simulink model "Pacemaker_model_assgn2_2019a"  (R2019a)
settings: Solver=FixedStepAuto  StartTime=0.0  StopTime=inf  FixedStep=1e-3  RelTol=1e-3  EnableMultiTasking=on
undefined symbols (not defined in the file): D0, D1, D10, D11, D12, D13, D2, D3, D4, D5, D6, D7, D8, D9, PTA0, PTA1, PTA2, PTB23, PTB9, PTC16, PTC17, PTC2, PTC3, PTC4, PTD0, PTD1, PTD2, PTD3
libraries: frdmk64flib x21, etargetslib x15, dspstat3 x1
settings Model: ExtModeTrigDuration=5  Creator=dr_pa  LastModifiedBy=dr_pa
settings SolverCC: ConcurrentTasks=on
settings OptimizationCC: EnhancedBackFolding=on  PassReuseOutputArgsAs=Individual arguments  MaxStackSize=64  OptimizeBlockOrder=speed  DifferentSizesBufferReuse=on  OptimizationCustomize=off
settings DebuggingCC: ParameterTunabilityLossMsg=error
settings HardwareCC: ProdBitPerPointer=32  ProdBitPerSizeT=32  ProdBitPerPtrDiffT=32  ProdLargestAtomicInteger=Long  ProdLargestAtomicFloat=Double  ProdWordSize=32  ProdHWDeviceType=ARM Compatible->ARM Cortex
settings SFSimCC: MATLABDynamicMemAlloc=off
settings RTWCC: SystemTargetFile=ert.tlc  HardwareBoard=NXP FRDM-K64F  TLCOptions="-aInlineSetEventsForThisBaseRateFcn=TLC_FALSE -aSuppressMultiTaskScheduler=TLC_FALSE  -aRateBasedStepFcn=0"  TemplateMakefile=ert_default_tmf  GenerateReport=on  Toolchain=GNU Tools for ARM Embedded Processors  BuildConfiguration=Faster Runs  IncludeHyperlinkInReport=on  LaunchReport=on  GenerateTraceInfo=on  GenerateTraceReport=on  GenerateTraceReportSl=on  GenerateTraceReportSf=on  GenerateTraceReportEml=on
settings CodeAppCC: ForceParamTrailComments=on  IgnoreCustomStorageClasses=off  OperatorAnnotations=on  SimulinkDataObjDesc=on  SFDataObjDesc=on  InsertBlockDesc=on

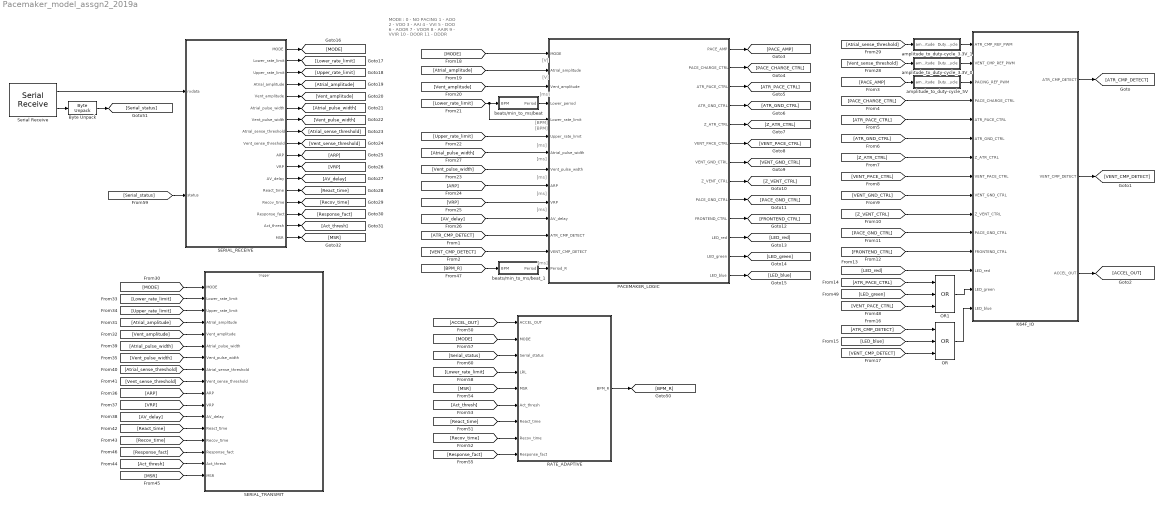
== system Pacemaker_model_assgn2_2019a ==
  note: [V]
  note: MODE :
      | 0 - NO PACING
      | 1 - AOO
      | 2 - VOO
      | 3 - AAI
      | 4 - VVI
      | 5 - DOO
      | 6 - AOOR
      | 7 - VOOR
      | 8 - AAIR
      | 9 - VVIR
      | 10 - DOOR
      | 11 - DDDR
  note: [V]
  note: [ms]
  note: [BPM]
  note: [BPM]
  note: [ms]
  note: [ms]
  note: [ms]
  note: [ms]
  note: [ms]
  note: [ms]
  Byte Unpack : etargetslib/Byte Unpack  dimensions={[1]}  datatypes={'uint8'}  byteAlign=1
      settings: SourceProductName=MATLAB Coder
  K64F_IO : Subsystem
  OR : Logic  Operator=OR  Inputs=3  IconShape=distinctive  AllPortsSameDT=off  OutDataTypeStr=boolean
  OR1 : Logic  Operator=OR  Inputs=3  IconShape=distinctive  AllPortsSameDT=off  OutDataTypeStr=boolean
  PACEMAKER_LOGIC : Stateflow chart  BlockKeywords=__PRM__SERIALIZED__DATA__:Stateflow Chart,Stateflow Diagram  TreatAsAtomicUnit=on
  RATE_ADAPTIVE : Subsystem
  SERIAL_RECEIVE : Stateflow chart  BlockKeywords=__PRM__SERIALIZED__DATA__:Stateflow Chart,Stateflow Diagram  TreatAsAtomicUnit=on
  SERIAL_TRANSMIT : Subsystem  TreatAsAtomicUnit=on
  Serial Receive : frdmk64flib/Serial Receive  SCIModule=0  Baudrate=uint32(9600)  Parity=None  StopBits=1  HardwareFlowControl=None  ByteOrder=LittleEndian  DataType=uint8  DataLength=56  BlockingMode=off  OutputStatus=on  SampleTime=-1
      settings: SourceProductName=Simulink Coder Support Package for NXP FRDM-K64F Board
  amplitude_to_duty-cycle_3.3V_0 : Subsystem
  amplitude_to_duty-cycle_3.3V_1 : Subsystem
  amplitude_to_duty-cycle_5V : Subsystem
  beats/min_to_ms/beat : Subsystem
  beats/min_to_ms/beat_1 : Subsystem
  wires:
  amplitude_to_duty-cycle_5V/1(Duty Cycle) -> K64F_IO/3(PACING_REF_PWM)
  beats/min_to_ms/beat/1(Period) -> PACEMAKER_LOGIC/4(Lower_period)
  amplitude_to_duty-cycle_3.3V_0/1(Duty Cycle) -> K64F_IO/2(VENT_CMP_REF_PWM)
  amplitude_to_duty-cycle_3.3V_1/1(Duty Cycle) -> K64F_IO/1(ATR_CMP_REF_PWM)
  K64F_IO/1(ATR_CMP_DETECT) -> [ATR_CMP_DETECT]
  [ATR_CMP_DETECT] -> PACEMAKER_LOGIC/12(ATR_CMP_DETECT)
  K64F_IO/2(VENT_CMP_DETECT) -> [VENT_CMP_DETECT]
  [VENT_CMP_DETECT] -> PACEMAKER_LOGIC/13(VENT_CMP_DETECT)
  K64F_IO/3(ACCEL_OUT) -> [ACCEL_OUT]
  RATE_ADAPTIVE/1(BPM_R) -> [BPM_R]
  OR/1 -> K64F_IO/15(LED_blue)
  Serial Receive/1 -> SERIAL_RECEIVE/1(rxdata)
  Serial Receive/2 -> Byte Unpack/1
  PACEMAKER_LOGIC/1(PACE_AMP) -> [PACE_AMP]
  [PACE_AMP] -> amplitude_to_duty-cycle_5V/1(amplitude)
  PACEMAKER_LOGIC/2(PACE_CHARGE_CTRL) -> [PACE_CHARGE_CTRL]
  [PACE_CHARGE_CTRL] -> K64F_IO/4(PACE_CHARGE_CTRL)
  [ATR_PACE_CTRL] -> K64F_IO/5(ATR_PACE_CTRL)
  PACEMAKER_LOGIC/4(ATR_GND_CTRL) -> [ATR_GND_CTRL]
  [ATR_GND_CTRL] -> K64F_IO/6(ATR_GND_CTRL)
  [Z_ATR_CTRL] -> K64F_IO/7(Z_ATR_CTRL)
  PACEMAKER_LOGIC/5(Z_ATR_CTRL) -> [Z_ATR_CTRL]
  PACEMAKER_LOGIC/6(VENT_PACE_CTRL) -> [VENT_PACE_CTRL]
  [VENT_PACE_CTRL] -> K64F_IO/8(VENT_PACE_CTRL)
  PACEMAKER_LOGIC/7(VENT_GND_CTRL) -> [VENT_GND_CTRL]
  [VENT_GND_CTRL] -> K64F_IO/9(VENT_GND_CTRL)
  PACEMAKER_LOGIC/8(Z_VENT_CTRL) -> [Z_VENT_CTRL]
  [Z_VENT_CTRL] -> K64F_IO/10(Z_VENT_CTRL)
  PACEMAKER_LOGIC/9(PACE_GND_CTRL) -> [PACE_GND_CTRL]
  [PACE_GND_CTRL] -> K64F_IO/11(PACE_GND_CTRL)
  [FRONTEND_CTRL] -> K64F_IO/12(FRONTEND_CTRL)
  PACEMAKER_LOGIC/10(FRONTEND_CTRL) -> [FRONTEND_CTRL]
  PACEMAKER_LOGIC/11(LED_red) -> [LED_red]
  [LED_red] -> K64F_IO/13(LED_red)
  PACEMAKER_LOGIC/12(LED_green) -> [LED_green]
  PACEMAKER_LOGIC/13(LED_blue) -> [LED_blue]
  [LED_blue] -> OR/2
  [ATR_CMP_DETECT] -> OR/1
  [VENT_CMP_DETECT] -> OR/3
  SERIAL_RECEIVE/1(MODE) -> [MODE]
  SERIAL_RECEIVE/2(Lower_rate_limit) -> [Lower_rate_limit]
  [AV_delay] -> PACEMAKER_LOGIC/11(AV_delay)
  [VRP] -> PACEMAKER_LOGIC/10(VRP)
  [ARP] -> PACEMAKER_LOGIC/9(ARP)
  [Vent_pulse_width] -> PACEMAKER_LOGIC/8(Vent_pulse_width)
  [Atrial_pulse_width] -> PACEMAKER_LOGIC/7(Atrial_pulse_width)
  [Upper_rate_limit] -> PACEMAKER_LOGIC/6(Upper_rate_limit)
  [Vent_amplitude] -> PACEMAKER_LOGIC/3(Vent_amplitude)
  [Atrial_amplitude] -> PACEMAKER_LOGIC/2(Atrial_amplitude)
  [MODE] -> PACEMAKER_LOGIC/1(MODE)
  [Lower_rate_limit] -> beats/min_to_ms/beat/1(BPM), PACEMAKER_LOGIC/5(Lower_rate_limit)
  SERIAL_RECEIVE/3(Upper_rate_limit) -> [Upper_rate_limit]
  SERIAL_RECEIVE/4(Atrial_amplitude) -> [Atrial_amplitude]
  SERIAL_RECEIVE/5(Vent_amplitude) -> [Vent_amplitude]
  SERIAL_RECEIVE/6(Atrial_pulse_width) -> [Atrial_pulse_width]
  SERIAL_RECEIVE/7(Vent_pulse_width) -> [Vent_pulse_width]
  SERIAL_RECEIVE/8(Atrial_sense_threshold) -> [Atrial_sense_threshold]
  SERIAL_RECEIVE/9(Vent_sense_threshold) -> [Vent_sense_threshold]
  SERIAL_RECEIVE/10(ARP) -> [ARP]
  SERIAL_RECEIVE/11(VRP) -> [VRP]
  SERIAL_RECEIVE/12(AV_delay) -> [AV_delay]
  SERIAL_RECEIVE/13(React_time) -> [React_time]
  SERIAL_RECEIVE/14(Recov_time) -> [Recov_time]
  SERIAL_RECEIVE/15(Response_fact) -> [Response_fact]
  SERIAL_RECEIVE/16(Act_thresh) -> [Act_thresh]
  SERIAL_RECEIVE/17(MSR) -> [MSR]
  [Vent_sense_threshold] -> amplitude_to_duty-cycle_3.3V_0/1(amplitude)
  [Atrial_sense_threshold] -> amplitude_to_duty-cycle_3.3V_1/1(amplitude)
  [MODE] -> SERIAL_TRANSMIT/1(MODE)
  [Atrial_amplitude] -> SERIAL_TRANSMIT/4(Atrial_amplitude)
  [Vent_amplitude] -> SERIAL_TRANSMIT/5(Vent_amplitude)
  [Lower_rate_limit] -> SERIAL_TRANSMIT/2(Lower_rate_limit)
  [Upper_rate_limit] -> SERIAL_TRANSMIT/3(Upper_rate_limit)
  [Atrial_pulse_width] -> SERIAL_TRANSMIT/6(Atrial_pulse_width)
  [Vent_pulse_width] -> SERIAL_TRANSMIT/7(Vent_pulse_width)
  [ARP] -> SERIAL_TRANSMIT/10(ARP)
  [VRP] -> SERIAL_TRANSMIT/11(VRP)
  [AV_delay] -> SERIAL_TRANSMIT/12(AV_delay)
  [Atrial_sense_threshold] -> SERIAL_TRANSMIT/8(Atrial_sense_threshold)
  [Vent_sense_threshold] -> SERIAL_TRANSMIT/9(Vent_sense_threshold)
  [React_time] -> SERIAL_TRANSMIT/13(React_time)
  [Recov_time] -> SERIAL_TRANSMIT/14(Recov_time)
  [MSR] -> SERIAL_TRANSMIT/17(MSR)
  [Act_thresh] -> SERIAL_TRANSMIT/16(Act_thresh)
  [Response_fact] -> SERIAL_TRANSMIT/15(Response_fact)
  beats/min_to_ms/beat_1/1(Period) -> PACEMAKER_LOGIC/14(Period_R)
  OR1/1 -> K64F_IO/14(LED_green)
  [ATR_PACE_CTRL] -> OR1/1
  [VENT_PACE_CTRL] -> OR1/3
  [LED_green] -> OR1/2
  [ACCEL_OUT] -> RATE_ADAPTIVE/1(ACCEL_OUT)
  [React_time] -> RATE_ADAPTIVE/7(React_time)
  [Recov_time] -> RATE_ADAPTIVE/8(Recov_time)
  [Response_fact] -> RATE_ADAPTIVE/9(Response_fact)
  [Act_thresh] -> RATE_ADAPTIVE/6(Act_thresh)
  [MSR] -> RATE_ADAPTIVE/5(MSR)
  [BPM_R] -> beats/min_to_ms/beat_1/1(BPM)
  [MODE] -> RATE_ADAPTIVE/2(MODE)
  [Lower_rate_limit] -> RATE_ADAPTIVE/4(LRL)
  PACEMAKER_LOGIC/3(ATR_PACE_CTRL) -> [ATR_PACE_CTRL]
  Byte Unpack/1 -> [Serial_status]
  [Serial_status] -> SERIAL_RECEIVE/2(status)
  [Serial_status] -> RATE_ADAPTIVE/3(Serial_status)

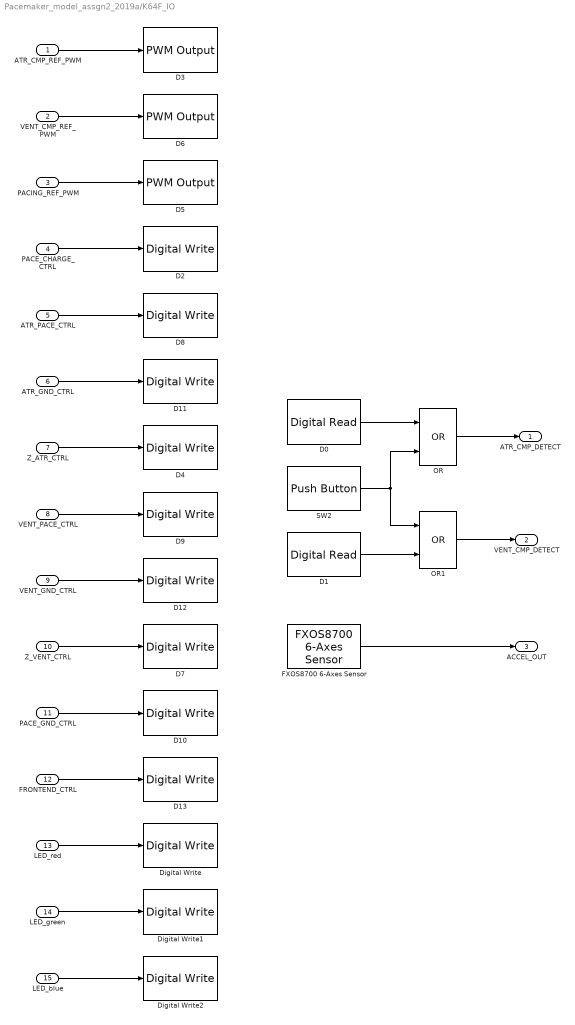
== system Pacemaker_model_assgn2_2019a/K64F_IO ==
  ATR_CMP_REF_PWM : Inport  OutDataTypeStr=uint8
  VENT_CMP_REF_PWM : Inport  Port=2  OutDataTypeStr=uint8
  PACING_REF_PWM : Inport  Port=3  OutDataTypeStr=uint8
  PACE_CHARGE_CTRL : Inport  Port=4  OutDataTypeStr=boolean
  ATR_PACE_CTRL : Inport  Port=5  OutDataTypeStr=boolean
  ATR_GND_CTRL : Inport  Port=6  OutDataTypeStr=boolean
  Z_ATR_CTRL : Inport  Port=7  OutDataTypeStr=boolean
  VENT_PACE_CTRL : Inport  Port=8  OutDataTypeStr=boolean
  VENT_GND_CTRL : Inport  Port=9  OutDataTypeStr=boolean
  Z_VENT_CTRL : Inport  Port=10  OutDataTypeStr=boolean
  PACE_GND_CTRL : Inport  Port=11  OutDataTypeStr=boolean
  FRONTEND_CTRL : Inport  Port=12  OutDataTypeStr=boolean
  LED_red : Inport  Port=13  OutDataTypeStr=boolean
  LED_green : Inport  Port=14  OutDataTypeStr=boolean
  LED_blue : Inport  Port=15  OutDataTypeStr=boolean
  D0 : frdmk64flib/Digital Read  Whichpin=PTC16 (D0)  SampleTime=-1
      settings: SourceProductName=Simulink Coder Support Package for NXP FRDM-K64F Board
  D1 : frdmk64flib/Digital Read  Whichpin=PTC17 (D1)  SampleTime=-1
      settings: SourceProductName=Simulink Coder Support Package for NXP FRDM-K64F Board
  D10 : frdmk64flib/Digital Write  Whichpin=PTD0 (D10)
      settings: SourceProductName=Simulink Coder Support Package for NXP FRDM-K64F Board
  D11 : frdmk64flib/Digital Write  Whichpin=PTD2 (D11)
      settings: SourceProductName=Simulink Coder Support Package for NXP FRDM-K64F Board
  D12 : frdmk64flib/Digital Write  Whichpin=PTD3 (D12)
      settings: SourceProductName=Simulink Coder Support Package for NXP FRDM-K64F Board
  D13 : frdmk64flib/Digital Write  Whichpin=PTD1 (D13)
      settings: SourceProductName=Simulink Coder Support Package for NXP FRDM-K64F Board
  D2 : frdmk64flib/Digital Write  Whichpin=PTB9 (D2)
      settings: SourceProductName=Simulink Coder Support Package for NXP FRDM-K64F Board
  D3 : frdmk64flib/PWM Output  Whichpin=PTA1 (D3)  InitialFrequency=2000  InitialDutyCycle=0
      settings: SourceProductName=Simulink Coder Support Package for NXP FRDM-K64F Board
  D4 : frdmk64flib/Digital Write  Whichpin=PTB23 (D4)
      settings: SourceProductName=Simulink Coder Support Package for NXP FRDM-K64F Board
  D5 : frdmk64flib/PWM Output  Whichpin=PTA2 (D5)  InitialFrequency=2000  InitialDutyCycle=0
      settings: SourceProductName=Simulink Coder Support Package for NXP FRDM-K64F Board
  D6 : frdmk64flib/PWM Output  Whichpin=PTC2 (D6)  InitialFrequency=2000  InitialDutyCycle=0
      settings: SourceProductName=Simulink Coder Support Package for NXP FRDM-K64F Board
  D7 : frdmk64flib/Digital Write  Whichpin=PTC3 (D7)
      settings: SourceProductName=Simulink Coder Support Package for NXP FRDM-K64F Board
  D8 : frdmk64flib/Digital Write  Whichpin=PTA0 (D8)
      settings: SourceProductName=Simulink Coder Support Package for NXP FRDM-K64F Board
  D9 : frdmk64flib/Digital Write  Whichpin=PTC4 (D9)
      settings: SourceProductName=Simulink Coder Support Package for NXP FRDM-K64F Board
  Digital Write : frdmk64flib/Digital Write  Whichpin=RED_LED
      settings: SourceProductName=Simulink Coder Support Package for NXP FRDM-K64F Board
  Digital Write1 : frdmk64flib/Digital Write  Whichpin=GREEN_LED
      settings: SourceProductName=Simulink Coder Support Package for NXP FRDM-K64F Board
  Digital Write2 : frdmk64flib/Digital Write  Whichpin=BLUE_LED
      settings: SourceProductName=Simulink Coder Support Package for NXP FRDM-K64F Board
  FXOS8700 6-Axes Sensor : frdmk64flib/FXOS8700 6-Axes Sensor  Activesensor=Accelerometer only  ODR=200Hz  HybridODR=100Hz  Accelfullrange=-4g to +4g  SampleTime=10e-3
      settings: SourceProductName=Simulink Coder Support Package for NXP FRDM-K64F Board
  OR : Logic  Operator=OR  IconShape=distinctive  AllPortsSameDT=off  OutDataTypeStr=boolean
  OR1 : Logic  Operator=OR  IconShape=distinctive  AllPortsSameDT=off  OutDataTypeStr=boolean
  SW2 : frdmk64flib/Push Button  Whichswitch=SW2  SampleTime1=-1
      settings: SourceProductName=Simulink Coder Support Package for NXP FRDM-K64F Board
  ATR_CMP_DETECT : Outport  OutDataTypeStr=boolean
  VENT_CMP_DETECT : Outport  Port=2  OutDataTypeStr=boolean
  ACCEL_OUT : Outport  Port=3  OutDataTypeStr=double
  wires:
  PACING_REF_PWM/1 -> D5/1
  PACE_CHARGE_CTRL/1 -> D2/1
  VENT_PACE_CTRL/1 -> D9/1
  VENT_GND_CTRL/1 -> D12/1
  ATR_PACE_CTRL/1 -> D8/1
  ATR_GND_CTRL/1 -> D11/1
  PACE_GND_CTRL/1 -> D10/1
  Z_ATR_CTRL/1 -> D4/1
  Z_VENT_CTRL/1 -> D7/1
  FRONTEND_CTRL/1 -> D13/1
  ATR_CMP_REF_PWM/1 -> D3/1
  VENT_CMP_REF_PWM/1 -> D6/1
  LED_red/1 -> Digital Write/1
  LED_green/1 -> Digital Write1/1
  D0/1 -> OR/1
  D1/1 -> OR1/2
  SW2/1 -> OR/2, OR1/1
  OR/1 -> ATR_CMP_DETECT/1
  OR1/1 -> VENT_CMP_DETECT/1
  LED_blue/1 -> Digital Write2/1
  FXOS8700 6-Axes Sensor/1 -> ACCEL_OUT/1

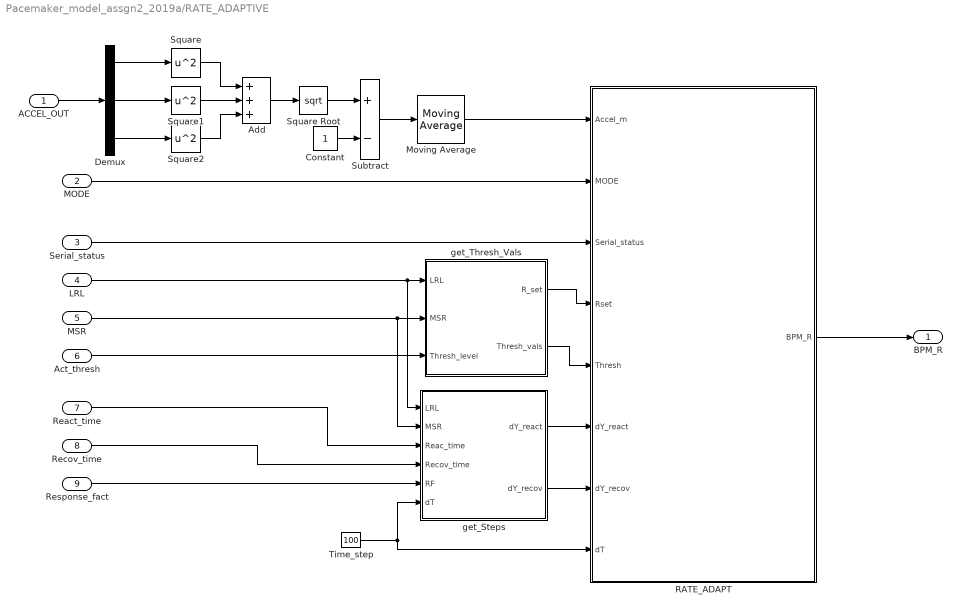
== system Pacemaker_model_assgn2_2019a/RATE_ADAPTIVE ==
  ACCEL_OUT : Inport  OutDataTypeStr=double
  MODE : Inport  Port=2  OutDataTypeStr=uint8
  Serial_status : Inport  Port=3  OutDataTypeStr=uint8
  LRL : Inport  Port=4  OutDataTypeStr=uint16
  MSR : Inport  Port=5  OutDataTypeStr=uint16
  Act_thresh : Inport  Port=6  OutDataTypeStr=uint8
  React_time : Inport  Port=7  OutDataTypeStr=uint16
  Recov_time : Inport  Port=8  OutDataTypeStr=uint16
  Response_fact : Inport  Port=9  OutDataTypeStr=uint8
  Add : Sum  Inputs=+++  AccumDataTypeStr=double  OutDataTypeStr=double
  Constant : Constant  OutDataTypeStr=double
  Demux : Demux  Outputs=3
  Moving Average : dspstat3/Moving Average  Method=Sliding window  ForgettingFactorPort=off  SpecifyWindowLength=on  WindowLength=25  ForgettingFactor=0.9  SimulateUsing=Code generation
  RATE_ADAPT : Stateflow chart  BlockKeywords=__PRM__SERIALIZED__DATA__:Stateflow Chart,Stateflow Diagram  TreatAsAtomicUnit=on
  Square : Math  Operator=square  OutDataTypeStr=double  SaturateOnIntegerOverflow=on
  Square Root : Sqrt  OutDataTypeStr=double  IntermediateResultsDataTypeStr=double  SaturateOnIntegerOverflow=on
  Square1 : Math  Operator=square  OutDataTypeStr=double  SaturateOnIntegerOverflow=on
  Square2 : Math  Operator=square  OutDataTypeStr=double  SaturateOnIntegerOverflow=on
  Subtract : Sum  Inputs=+-
  Time_step : Constant  Value=100  OutDataTypeStr=uint16
  get_Steps : Subsystem
  get_Thresh_Vals : Subsystem
  BPM_R : Outport  OutDataTypeStr=double
  wires:
  get_Steps/1(dY_react) -> RATE_ADAPT/6(dY_react)
  get_Steps/2(dY_recov) -> RATE_ADAPT/7(dY_recov)
  Response_fact/1 -> get_Steps/5(RF)
  Demux/1 -> Square/1
  Time_step/1 -> get_Steps/6(dT), RATE_ADAPT/8(dT)
  Square2/1 -> Add/3
  Moving Average/1 -> RATE_ADAPT/1(Accel_m)
  Square/1 -> Add/1
  Square1/1 -> Add/2
  ACCEL_OUT/1 -> Demux/1
  Constant/1 -> Subtract/2
  MSR/1 -> get_Thresh_Vals/2(MSR), get_Steps/2(MSR)
  LRL/1 -> get_Thresh_Vals/1(LRL), get_Steps/1(LRL)
  Subtract/1 -> Moving Average/1
  Act_thresh/1 -> get_Thresh_Vals/3(Thresh_level)
  Recov_time/1 -> get_Steps/4(Recov_time)
  get_Thresh_Vals/1(R_set) -> RATE_ADAPT/4(Rset)
  get_Thresh_Vals/2(Thresh_vals) -> RATE_ADAPT/5(Thresh)
  Square Root/1 -> Subtract/1
  RATE_ADAPT/1(BPM_R) -> BPM_R/1
  Demux/2 -> Square1/1
  Demux/3 -> Square2/1
  Add/1 -> Square Root/1
  MODE/1 -> RATE_ADAPT/2(MODE)
  React_time/1 -> get_Steps/3(Reac_time)
  Serial_status/1 -> RATE_ADAPT/3(Serial_status)

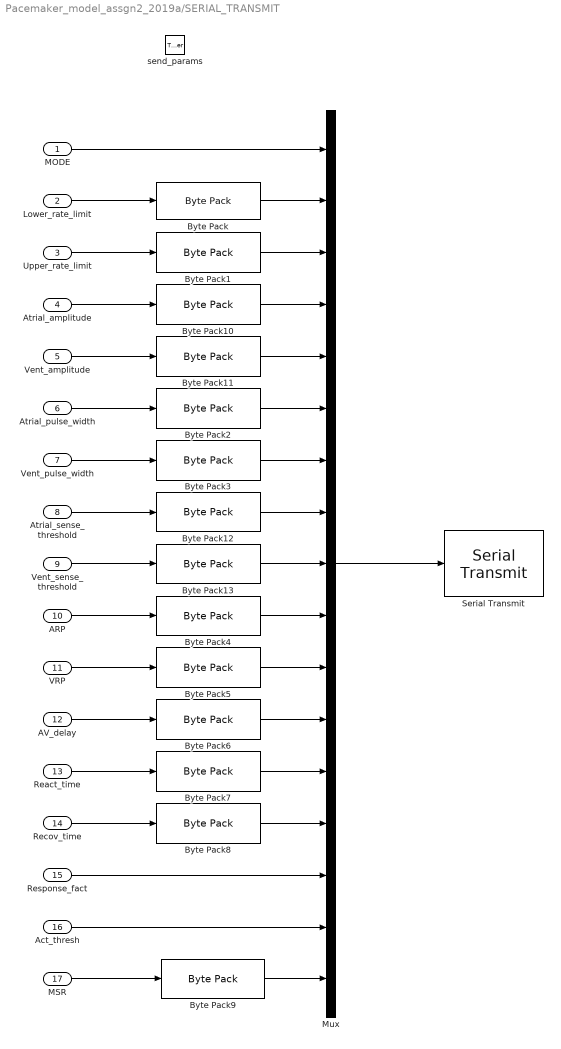
== system Pacemaker_model_assgn2_2019a/SERIAL_TRANSMIT ==
  MODE : Inport
  Lower_rate_limit : Inport  Port=2
  Upper_rate_limit : Inport  Port=3
  Atrial_amplitude : Inport  Port=4
  Vent_amplitude : Inport  Port=5
  Atrial_pulse_width : Inport  Port=6
  Vent_pulse_width : Inport  Port=7
  Atrial_sense_threshold : Inport  Port=8
  Vent_sense_threshold : Inport  Port=9
  ARP : Inport  Port=10
  VRP : Inport  Port=11
  AV_delay : Inport  Port=12
  React_time : Inport  Port=13
  Recov_time : Inport  Port=14
  Response_fact : Inport  Port=15
  Act_thresh : Inport  Port=16
  MSR : Inport  Port=17
  send_params : TriggerPort  TriggerType=function-call  IsSimulinkFunction=on  FunctionName=send_params  VariantControl=Variant
  Byte Pack{,1..9} (10 alike) : etargetslib/Byte Pack  datatypes={'uint16'}  byteAlign=1
      settings: SourceProductName=MATLAB Coder
  Byte Pack{10..13} (4 alike) : etargetslib/Byte Pack  datatypes={'double'}  byteAlign=1
      settings: SourceProductName=MATLAB Coder
  Mux : Mux  Inputs=17
  Serial Transmit : frdmk64flib/Serial Transmit  SCIModule=0  Baudrate=uint32(9600)  Parity=None  StopBits=1  HardwareFlowControl=None  ByteOrder=LittleEndian  BlockingMode=on  OutputStatus=off
      settings: SourceProductName=Simulink Coder Support Package for NXP FRDM-K64F Board
  wires:
  MSR/1 -> Byte Pack9/1
  AV_delay/1 -> Byte Pack6/1
  VRP/1 -> Byte Pack5/1
  Recov_time/1 -> Byte Pack8/1
  Vent_sense_threshold/1 -> Byte Pack13/1
  ARP/1 -> Byte Pack4/1
  Upper_rate_limit/1 -> Byte Pack1/1
  Vent_amplitude/1 -> Byte Pack11/1
  Atrial_amplitude/1 -> Byte Pack10/1
  React_time/1 -> Byte Pack7/1
  Atrial_pulse_width/1 -> Byte Pack2/1
  Atrial_sense_threshold/1 -> Byte Pack12/1
  Lower_rate_limit/1 -> Byte Pack/1
  Vent_pulse_width/1 -> Byte Pack3/1
  Response_fact/1 -> Mux/15
  Act_thresh/1 -> Mux/16
  Byte Pack9/1 -> Mux/17
  Byte Pack8/1 -> Mux/14
  Byte Pack7/1 -> Mux/13
  Byte Pack6/1 -> Mux/12
  Byte Pack5/1 -> Mux/11
  Byte Pack4/1 -> Mux/10
  Byte Pack13/1 -> Mux/9
  Byte Pack12/1 -> Mux/8
  Byte Pack3/1 -> Mux/7
  Byte Pack2/1 -> Mux/6
  Byte Pack11/1 -> Mux/5
  Byte Pack10/1 -> Mux/4
  Byte Pack1/1 -> Mux/3
  MODE/1 -> Mux/1
  Byte Pack/1 -> Mux/2
  Mux/1 -> Serial Transmit/1

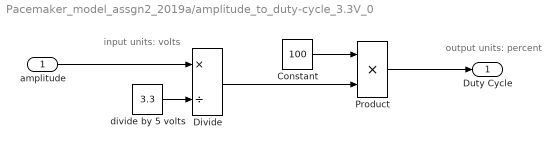
== system Pacemaker_model_assgn2_2019a/amplitude_to_duty-cycle_3.3V_0 ==
  note: input units: volts
  note: output units: percent
  amplitude : Inport  OutDataTypeStr=double
  Constant : Constant  Value=100  OutDataTypeStr=double
  Divide : Product  Inputs=*/  OutDataTypeStr=double
  Product : Product  OutDataTypeStr=uint8  RndMeth=Round
  divide by 5 volts : Constant  Value=3.3  OutDataTypeStr=double
  Duty Cycle : Outport  OutDataTypeStr=uint8
  wires:
  amplitude/1 -> Divide/1
  Product/1 -> Duty Cycle/1
  Constant/1 -> Product/1
  Divide/1 -> Product/2
  divide by 5 volts/1 -> Divide/2

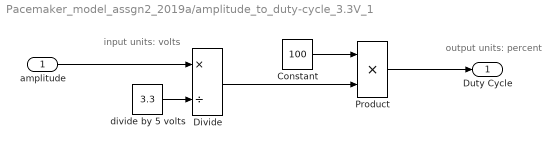
== system Pacemaker_model_assgn2_2019a/amplitude_to_duty-cycle_3.3V_1 ==
  note: output units: percent
  note: input units: volts
  amplitude : Inport  OutDataTypeStr=double
  Constant : Constant  Value=100  OutDataTypeStr=double
  Divide : Product  Inputs=*/  OutDataTypeStr=double
  Product : Product  OutDataTypeStr=uint8  RndMeth=Round
  divide by 5 volts : Constant  Value=3.3  OutDataTypeStr=double
  Duty Cycle : Outport  OutDataTypeStr=uint8
  wires:
  divide by 5 volts/1 -> Divide/2
  Divide/1 -> Product/2
  Constant/1 -> Product/1
  Product/1 -> Duty Cycle/1
  amplitude/1 -> Divide/1

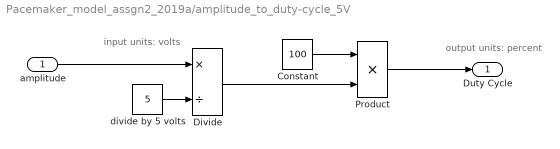
== system Pacemaker_model_assgn2_2019a/amplitude_to_duty-cycle_5V ==
  note: output units: percent
  note: input units: volts
  amplitude : Inport  OutDataTypeStr=double
  Constant : Constant  Value=100  OutDataTypeStr=double
  Divide : Product  Inputs=*/  OutDataTypeStr=double
  Product : Product  OutDataTypeStr=uint8  RndMeth=Round
  divide by 5 volts : Constant  Value=5  OutDataTypeStr=double
  Duty Cycle : Outport  OutDataTypeStr=uint8
  wires:
  divide by 5 volts/1 -> Divide/2
  Divide/1 -> Product/2
  Constant/1 -> Product/1
  Product/1 -> Duty Cycle/1
  amplitude/1 -> Divide/1

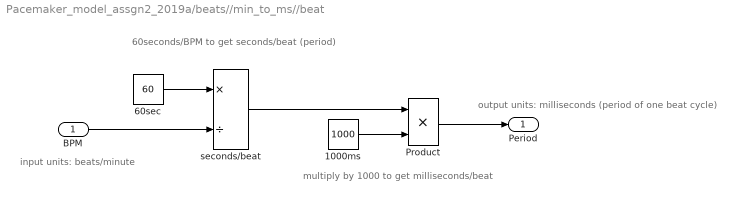
== system Pacemaker_model_assgn2_2019a/beats//min_to_ms//beat ==
  note: input units: beats/minute
  note: output units: milliseconds (period of one beat cycle)
  note: 60seconds/BPM to get seconds/beat (period)
  note: multiply by 1000 to get milliseconds/beat
  BPM : Inport  OutDataTypeStr=uint16
  1000ms : Constant  Value=1000  OutDataTypeStr=double
  60sec : Constant  Value=60  OutDataTypeStr=double
  Product : Product  OutDataTypeStr=uint16  RndMeth=Round
  seconds/beat : Product  Inputs=*/  OutDataTypeStr=double
  Period : Outport  OutDataTypeStr=uint16
  wires:
  1000ms/1 -> Product/2
  Product/1 -> Period/1
  seconds/beat/1 -> Product/1
  60sec/1 -> seconds/beat/1
  BPM/1 -> seconds/beat/2

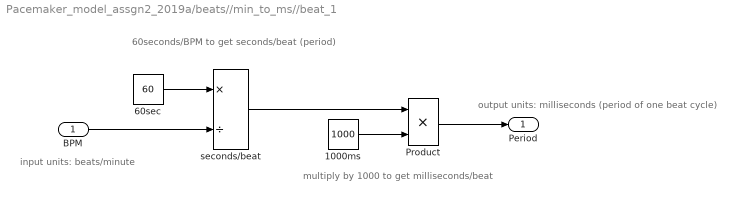
== system Pacemaker_model_assgn2_2019a/beats//min_to_ms//beat_1 ==
  note: input units: beats/minute
  note: output units: milliseconds (period of one beat cycle)
  note: 60seconds/BPM to get seconds/beat (period)
  note: multiply by 1000 to get milliseconds/beat
  BPM : Inport  OutDataTypeStr=double
  1000ms : Constant  Value=1000  OutDataTypeStr=double
  60sec : Constant  Value=60  OutDataTypeStr=double
  Product : Product  OutDataTypeStr=uint16  RndMeth=Round
  seconds/beat : Product  Inputs=*/  OutDataTypeStr=double
  Period : Outport  OutDataTypeStr=uint16
  wires:
  1000ms/1 -> Product/2
  Product/1 -> Period/1
  seconds/beat/1 -> Product/1
  60sec/1 -> seconds/beat/1
  BPM/1 -> seconds/beat/2

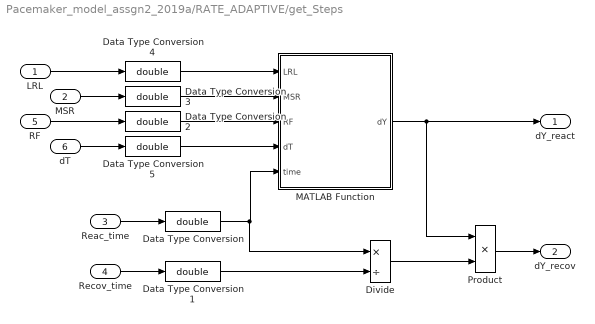
== system Pacemaker_model_assgn2_2019a/RATE_ADAPTIVE/get_Steps ==
  LRL : Inport  OutDataTypeStr=uint16
  MSR : Inport  Port=2  OutDataTypeStr=uint16
  Reac_time : Inport  Port=3  OutDataTypeStr=uint16
  Recov_time : Inport  Port=4  OutDataTypeStr=uint16
  RF : Inport  Port=5  OutDataTypeStr=uint8
  dT : Inport  Port=6  OutDataTypeStr=uint16
  Data Type Conversion{,1..5} (6 alike) : DataTypeConversion  OutDataTypeStr=double
  Divide : Product  Inputs=*/
  MATLAB Function : MATLAB Function  TreatAsAtomicUnit=on
  Product : Product  OutDataTypeStr=double  RndMeth=Round
  dY_react : Outport  OutDataTypeStr=double
  dY_recov : Outport  Port=2  OutDataTypeStr=double
  wires:
  Reac_time/1 -> Data Type Conversion/1
  RF/1 -> Data Type Conversion2/1
  MATLAB Function/1(dY) -> Product/1, dY_react/1
  MSR/1 -> Data Type Conversion3/1
  LRL/1 -> Data Type Conversion4/1
  Data Type Conversion/1 -> Divide/1, MATLAB Function/5(time)
  Data Type Conversion4/1 -> MATLAB Function/1(LRL)
  Data Type Conversion3/1 -> MATLAB Function/2(MSR)
  Data Type Conversion2/1 -> MATLAB Function/3(RF)
  dT/1 -> Data Type Conversion5/1
  Data Type Conversion5/1 -> MATLAB Function/4(dT)
  Recov_time/1 -> Data Type Conversion1/1
  Product/1 -> dY_recov/1
  Data Type Conversion1/1 -> Divide/2
  Divide/1 -> Product/2

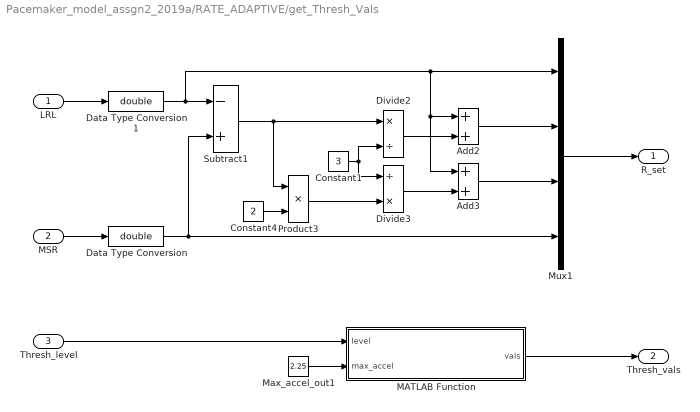
== system Pacemaker_model_assgn2_2019a/RATE_ADAPTIVE/get_Thresh_Vals ==
  LRL : Inport  OutDataTypeStr=uint16
  MSR : Inport  Port=2  OutDataTypeStr=uint16
  Thresh_level : Inport  Port=3  OutDataTypeStr=uint8
  Add2 : Sum  AccumDataTypeStr=double  OutDataTypeStr=double
  Add3 : Sum  AccumDataTypeStr=double  OutDataTypeStr=double
  Constant1 : Constant  Value=3  OutDataTypeStr=double
  Constant4 : Constant  Value=2  OutDataTypeStr=double
  Data Type Conversion : DataTypeConversion  OutDataTypeStr=double
  Data Type Conversion1 : DataTypeConversion  OutDataTypeStr=double
  Divide2 : Product  Inputs=*/  OutDataTypeStr=double
  Divide3 : Product  Inputs=/*  OutDataTypeStr=double
  MATLAB Function : MATLAB Function  TreatAsAtomicUnit=on
  Max_accel_out1 : Constant  Value=2.25  OutDataTypeStr=double
  Mux1 : Mux
  Product3 : Product  OutDataTypeStr=double
  Subtract1 : Sum  Inputs=-+  AccumDataTypeStr=double  OutDataTypeStr=double
  R_set : Outport  OutDataTypeStr=double
  Thresh_vals : Outport  Port=2  OutDataTypeStr=double
  wires:
  Mux1/1 -> R_set/1
  Subtract1/1 -> Product3/1, Divide2/1
  Constant4/1 -> Product3/2
  Constant1/1 -> Divide2/2, Divide3/1
  Product3/1 -> Divide3/2
  Divide3/1 -> Add3/2
  Divide2/1 -> Add2/2
  Add3/1 -> Mux1/3
  Add2/1 -> Mux1/2
  MSR/1 -> Data Type Conversion/1
  Data Type Conversion/1 -> Mux1/4, Subtract1/2
  LRL/1 -> Data Type Conversion1/1
  Data Type Conversion1/1 -> Add3/1, Add2/1, Mux1/1, Subtract1/1
  Max_accel_out1/1 -> MATLAB Function/2(max_accel)
  Thresh_level/1 -> MATLAB Function/1(level)
  MATLAB Function/1(vals) -> Thresh_vals/1

== stateflow chart Pacemaker_model_assgn2_2019a/RATE_ADAPTIVE/RATE_ADAPT ==
  state HIGH
    entry:
    if abs(Rset(4)-BPM_R)<1.0
    BPM_R = Rset(4);
    end
  state M_HIGH
    entry:
    if abs(Rset(3)-BPM_R)<1.0
    BPM_R = Rset(3);
    end
  state Init
    entry:
    BPM_R = Rset(1);
  state LOW
    entry:
    if abs(Rset(1)-BPM_R)<1.0
    BPM_R = Rset(1);
    end
  state M_LOW
    entry:
    if abs(Rset(2)-BPM_R)<1.0
    BPM_R = Rset(2);
    end
  M_HIGH -> (junction 51) [order 4] : [Serial_status==0]
  HIGH -> HIGH [order 2] : [after(dT,msec) && Rset(4)>BPM_R]
      | {BPM_R = BPM_R + dY_react}
  M_HIGH -> M_HIGH [order 3] : [after(dT,msec) && Rset(3)<BPM_R]
      | {BPM_R = BPM_R - dY_recov}
  M_HIGH -> M_HIGH [order 2] : [after(dT,msec) && Rset(3)>BPM_R]
      | {BPM_R = BPM_R + dY_react}
  HIGH -> (junction 51) [order 3] : [Serial_status==0]
  M_HIGH -> (junction 12) [order 1] : [Accel_m<Thresh(2) || Accel_m>Thresh(3)]
  (junction 12) -> M_HIGH [order 2] : [Accel_m>Thresh(2)]
  (junction 12) -> HIGH [order 1] : [Accel_m>Thresh(3)]
  HIGH -> (junction 12) [order 1] : [Accel_m<Thresh(3)]
  (default) -> Init
  (junction 51) -> Init
  Init -> (junction 12) : [MODE>=6]
  LOW -> (junction 51) [order 3] : [Serial_status==0]
  (junction 12) -> M_LOW [order 3] : [Accel_m>Thresh(1)]
  (junction 12) -> LOW [order 4] : [Accel_m>0]
  M_LOW -> (junction 51) [order 4] : [Serial_status==0]
  M_LOW -> (junction 12) [order 1] : [Accel_m<Thresh(1) || Accel_m>Thresh(2)]
  LOW -> (junction 12) [order 1] : [Accel_m>Thresh(1)]
  M_LOW -> M_LOW [order 2] : [after(dT,msec) && Rset(2)>BPM_R]
      | {BPM_R = BPM_R + dY_react}
  M_LOW -> M_LOW [order 3] : [after(dT,msec) && Rset(2)<BPM_R]
      | {BPM_R = BPM_R - dY_recov}
  LOW -> LOW [order 2] : [after(dT,msec) && Rset(1)<BPM_R]
      | {BPM_R = BPM_R - dY_recov}
  data: Accel_m input double; MODE input uint8; Serial_status input uint8; Rset input double; Thresh input double; dY_react input double; dY_recov input double; BPM_R output double; dT input uint16

== stateflow chart Pacemaker_model_assgn2_2019a/SERIAL_RECEIVE ==
  state PARAMETER_CHECK
    entry:
    if Lower_rate_limit < 50 || Lower_rate_limit > 175 || Upper_rate_limit < 75 || Upper_rate_limit > 175 ...
    || Atrial_amplitude < 0.5 || Atrial_amplitude > 5 || Vent_amplitude < 0.5 || Vent_amplitude > 5 ...
    || Atrial_pulse_width < 1 || Atrial_pulse_width > 10 || Vent_pulse_width < 1 || Vent_pulse_width > 10 ...
    || Atrial_sense_threshold < 0.5 || Atrial_sense_threshold > 3.3 || Vent_sense_threshold < 0.5 ...
    || Vent_sense_threshold > 3.3 || ARP < 150 || ARP > 500 || VRP < 150 || VRP > 500 || AV_delay < 70 ...
    || AV_delay > 300 || React_time < 1 || React_time > 30 || Recov_time < 5 || Recov_time > 30 ...
    || Response_fact < 1 || Response_fact > 16 || Act_thresh < 1 || Act_thresh > 4 || MSR < 50 || MSR > 175
    MODE = 0;   %move to safe state if parameters out of range
    end
  state SET_PARAMS
    %we assume this is the order that the data is sent in
    entry:
    MODE = rxdata(1);
    Lower_rate_limit = typecast(rxdata(2:3), 'uint16');
    Upper_rate_limit = typecast(rxdata(4:5), 'uint16');
    Atrial_amplitude = typecast(rxdata(6:13), 'double');
    Vent_amplitude = typecast(rxdata(14:21), 'double');
    Atrial_pulse_width = typecast(rxdata(22:23), 'uint16');
    Vent_pulse_width = typecast(rxdata(24:25), 'uint16')
    Atrial_sense_threshold = typecast(rxdata(26:33), 'double')
    Vent_sense_threshold = typecast(rxdata(34:41), 'double')
    ARP = typecast(rxdata(42:43), 'uint16')
    VRP = typecast(rxdata(44:45), 'uint16')
    AV_delay = typecast(rxdata(46:47), 'uint16')
    React_time = typecast(rxdata(48:49), 'uint16')
    Recov_time = typecast(rxdata(50:51), 'uint16')
    Response_fact = rxdata(52)
    Act_thresh = rxdata(53)
    MSR = typecast(rxdata(54:55), 'uint16')
    send_params();
  state INITIAL
    entry:
    MODE = 0;
    Lower_rate_limit = 60;
    Upper_rate_limit = 150;
    Atrial_amplitude = 3.3;
    Vent_amplitude = 3.3;
    Atrial_pulse_width = 10;
    Vent_pulse_width = 10;
    Atrial_sense_threshold = 2.75;
    Vent_sense_threshold = 2.75;
    ARP = 300;
    VRP = 300;
    AV_delay = 100;
    React_time = 4; %unknown
    Recov_time = 10; %unknown
    Response_fact = 8; %unknown
    Act_thresh = 1; %unknown
    MSR = 120; %unknown
  state STANDBY
    %Waiting for COM
  PARAMETER_CHECK -> STANDBY
  SET_PARAMS -> PARAMETER_CHECK
  (default) -> INITIAL
  INITIAL -> STANDBY
  STANDBY -> SET_PARAMS : [status == 0]
  data: rxdata input uint8; status input uint8; MODE output uint8; Lower_rate_limit output uint16; Upper_rate_limit output uint16; Atrial_amplitude output double; Vent_amplitude output double; Atrial_pulse_width output uint16; Vent_pulse_width output uint16; Atrial_sense_threshold output double; Vent_sense_threshold output double; ARP output uint16; VRP output uint16; AV_delay output uint16; React_time output uint16; Recov_time output uint16; Response_fact output uint8; Act_thresh output uint8; MSR output uint16

== stateflow chart Pacemaker_model_assgn2_2019a/PACEMAKER_LOGIC ==
  state AOOR [group]
    state AOOR_PACE_ATRIUM
      entry:
      PACE_CHARGE_CTRL = false;
      PACE_GND_CTRL = true;
      VENT_PACE_CTRL = false;
      VENT_GND_CTRL = false;
      Z_VENT_CTRL = false;
      Z_ATR_CTRL = false;
      ATR_GND_CTRL = false;
      ATR_PACE_CTRL = true;
    state AOOR_DischargeC21_ChargeC22
      entry:
      PACE_GND_CTRL = true;
      ATR_PACE_CTRL = false;
      Z_ATR_CTRL = false;
      Z_VENT_CTRL = false;
      VENT_PACE_CTRL = false;
      VENT_GND_CTRL = false;
      ATR_GND_CTRL = true;
      PACE_AMP = Atrial_amplitude;
      PACE_CHARGE_CTRL = true;
    AOOR_DischargeC21_ChargeC22 -> AOOR_PACE_ATRIUM [order 1] : after((Period_R-Atrial_pulse_width), msec)
    AOOR_PACE_ATRIUM -> AOOR_DischargeC21_ChargeC22 : after(Atrial_pulse_width, msec)
  state AOO [group]
    state AOO_PACE_ATRIUM
      entry:
      PACE_CHARGE_CTRL = false;
      PACE_GND_CTRL = true;
      VENT_PACE_CTRL = false;
      VENT_GND_CTRL = false;
      Z_VENT_CTRL = false;
      Z_ATR_CTRL = false;
      ATR_GND_CTRL = false;
      ATR_PACE_CTRL = true;
    state AOO_DischargeC21_ChargeC22
      entry:
      PACE_GND_CTRL = true;
      ATR_PACE_CTRL = false;
      Z_ATR_CTRL = false;
      Z_VENT_CTRL = false;
      VENT_PACE_CTRL = false;
      VENT_GND_CTRL = false;
      ATR_GND_CTRL = true;
      PACE_AMP = Atrial_amplitude;
      PACE_CHARGE_CTRL = true;
    AOO_DischargeC21_ChargeC22 -> AOO_PACE_ATRIUM [order 1] : after((Lower_period-Atrial_pulse_width), msec)
    AOO_PACE_ATRIUM -> AOO_DischargeC21_ChargeC22 : after(Atrial_pulse_width, msec)
  state VOOR [group]
    state VOOR_PACE_VENT
      entry:
      PACE_CHARGE_CTRL = false;
      PACE_GND_CTRL = true;
      ATR_PACE_CTRL = false;
      ATR_GND_CTRL = false;
      Z_ATR_CTRL = false;
      Z_VENT_CTRL = false;
      VENT_GND_CTRL = false;
      VENT_PACE_CTRL = true;
    state VOOR_DischargeC21_ChargeC22
      entry:
      PACE_GND_CTRL = true;
      VENT_PACE_CTRL = false;
      Z_VENT_CTRL = false;
      Z_ATR_CTRL = false;
      ATR_PACE_CTRL = false;
      ATR_GND_CTRL = false;
      VENT_GND_CTRL = true;
      PACE_AMP = Vent_amplitude;
      PACE_CHARGE_CTRL = true;
    VOOR_DischargeC21_ChargeC22 -> VOOR_PACE_VENT [order 1] : after((Period_R-Vent_pulse_width), msec)
    VOOR_PACE_VENT -> VOOR_DischargeC21_ChargeC22 : after(Vent_pulse_width, msec)
  state VOO [group]
    state VOO_PACE_VENT
      entry:
      PACE_CHARGE_CTRL = false;
      PACE_GND_CTRL = true;
      ATR_PACE_CTRL = false;
      ATR_GND_CTRL = false;
      Z_ATR_CTRL = false;
      Z_VENT_CTRL = false;
      VENT_GND_CTRL = false;
      VENT_PACE_CTRL = true;
    state VOO_DischargeC21_ChargeC22
      entry:
      PACE_GND_CTRL = true;
      VENT_PACE_CTRL = false;
      Z_VENT_CTRL = false;
      Z_ATR_CTRL = false;
      ATR_PACE_CTRL = false;
      ATR_GND_CTRL = false;
      VENT_GND_CTRL = true;
      PACE_AMP = Vent_amplitude;
      PACE_CHARGE_CTRL = true;
    VOO_DischargeC21_ChargeC22 -> VOO_PACE_VENT [order 1] : after((Lower_period-Vent_pulse_width), msec)
    VOO_PACE_VENT -> VOO_DischargeC21_ChargeC22 : after(Vent_pulse_width, msec)
  state AAI [group]
    state ARP
      entry:
      PACE_GND_CTRL = true;
      ATR_PACE_CTRL = false;
      Z_ATR_CTRL = false;
      Z_VENT_CTRL = false;
      VENT_PACE_CTRL = false;
      VENT_GND_CTRL = false;
      ATR_GND_CTRL = true;
      PACE_CHARGE_CTRL = true;
      FRONTEND_CTRL = true;
    state AAI_PACE_ATRIUM
      entry:
      PACE_CHARGE_CTRL = false;
      PACE_GND_CTRL = true;
      VENT_PACE_CTRL = false;
      VENT_GND_CTRL = false;
      Z_VENT_CTRL = false;
      Z_ATR_CTRL = false;
      ATR_GND_CTRL = false;
      FRONTEND_CTRL = false;
      ATR_PACE_CTRL = true;
      APW_delay = Atrial_pulse_width;
    state AAI_DischargeC21_ChargeC22
      entry:
      PACE_GND_CTRL = true;
      ATR_PACE_CTRL = false;
      Z_ATR_CTRL = false;
      Z_VENT_CTRL = false;
      VENT_PACE_CTRL = false;
      VENT_GND_CTRL = false;
      ATR_GND_CTRL = true;
      PACE_AMP = Atrial_amplitude;
      PACE_CHARGE_CTRL = true;
    AAI_PACE_ATRIUM -> AAI.ARP : after(Atrial_pulse_width, msec)
    AAI_DischargeC21_ChargeC22 -> AAI.ARP [order 1] : [ATR_CMP_DETECT==true]
        | {APW_delay = 0;}
    AAI.ARP -> AAI_DischargeC21_ChargeC22 : after(ARP, msec)
    AAI_DischargeC21_ChargeC22 -> AAI_PACE_ATRIUM [order 2] : after((Lower_period-ARP-APW_delay), msec)
  state AAIR [group]
    state ARP
      entry:
      PACE_GND_CTRL = true;
      ATR_PACE_CTRL = false;
      Z_ATR_CTRL = false;
      Z_VENT_CTRL = false;
      VENT_PACE_CTRL = false;
      VENT_GND_CTRL = false;
      ATR_GND_CTRL = true;
      PACE_CHARGE_CTRL = true;
      FRONTEND_CTRL = true;
    state AAIR_PACE_ATRIUM
      entry:
      PACE_CHARGE_CTRL = false;
      PACE_GND_CTRL = true;
      VENT_PACE_CTRL = false;
      VENT_GND_CTRL = false;
      Z_VENT_CTRL = false;
      Z_ATR_CTRL = false;
      ATR_GND_CTRL = false;
      FRONTEND_CTRL = false;
      ATR_PACE_CTRL = true;
      APW_delay = Atrial_pulse_width;
    state AAIR_DischargeC21_ChargeC22
      entry:
      PACE_GND_CTRL = true;
      ATR_PACE_CTRL = false;
      Z_ATR_CTRL = false;
      Z_VENT_CTRL = false;
      VENT_PACE_CTRL = false;
      VENT_GND_CTRL = false;
      ATR_GND_CTRL = true;
      PACE_AMP = Atrial_amplitude;
      PACE_CHARGE_CTRL = true;
    AAIR_PACE_ATRIUM -> AAIR.ARP : after(Atrial_pulse_width, msec)
    AAIR_DischargeC21_ChargeC22 -> AAIR.ARP [order 1] : [ATR_CMP_DETECT==true]
        | {APW_delay = 0;}
    AAIR.ARP -> AAIR_DischargeC21_ChargeC22 : after(ARP, msec)
    AAIR_DischargeC21_ChargeC22 -> AAIR_PACE_ATRIUM [order 2] : after((Period_R-ARP-APW_delay), msec)
  state STANDBY
    entry:
    PACE_CHARGE_CTRL = false;
    PACE_GND_CTRL = false;
    ATR_GND_CTRL = false;
    VENT_GND_CTRL = false;
    ATR_PACE_CTRL = false;
    VENT_PACE_CTRL = false;
    FRONTEND_CTRL = true;
    LED_red = true;
    LED_green = false;
    LED_blue = false;
    APW_delay = 0;
    VPW_delay = 0;
  state VVI [group]
    state VRP
      entry:
      PACE_GND_CTRL = true;
      VENT_PACE_CTRL = false;
      Z_VENT_CTRL = false;
      Z_ATR_CTRL = false;
      ATR_PACE_CTRL = false;
      ATR_GND_CTRL = false;
      VENT_GND_CTRL = true;
      PACE_CHARGE_CTRL = true;
      FRONTEND_CTRL = true;
    state VVI_PACE_VENT
      entry:
      PACE_CHARGE_CTRL = false;
      PACE_GND_CTRL = true;
      ATR_PACE_CTRL = false;
      ATR_GND_CTRL = false;
      Z_ATR_CTRL = false;
      Z_VENT_CTRL = false;
      VENT_GND_CTRL = false;
      FRONTEND_CTRL = false;
      VENT_PACE_CTRL = true;
      VPW_delay = Vent_pulse_width;
    state VVI_DischargeC21_ChargeC22
      entry:
      PACE_GND_CTRL = true;
      VENT_PACE_CTRL = false;
      Z_VENT_CTRL = false;
      Z_ATR_CTRL = false;
      ATR_PACE_CTRL = false;
      ATR_GND_CTRL = false;
      VENT_GND_CTRL = true;
      PACE_AMP = Vent_amplitude;
      PACE_CHARGE_CTRL = true;
    VVI_DischargeC21_ChargeC22 -> VVI.VRP [order 1] : [VENT_CMP_DETECT==true]
        | {VPW_delay = 0;}
    VVI_PACE_VENT -> VVI.VRP : after(Vent_pulse_width, msec)
    VVI.VRP -> VVI_DischargeC21_ChargeC22 : after(VRP, msec)
    VVI_DischargeC21_ChargeC22 -> VVI_PACE_VENT [order 2] : after(Lower_period-VRP-VPW_delay, msec)
  state VVIR [group]
    state VRP
      entry:
      PACE_GND_CTRL = true;
      VENT_PACE_CTRL = false;
      Z_VENT_CTRL = false;
      Z_ATR_CTRL = false;
      ATR_PACE_CTRL = false;
      ATR_GND_CTRL = false;
      VENT_GND_CTRL = true;
      PACE_CHARGE_CTRL = true;
      FRONTEND_CTRL = true;
    state VVIR_PACE_VENT
      entry:
      PACE_CHARGE_CTRL = false;
      PACE_GND_CTRL = true;
      ATR_PACE_CTRL = false;
      ATR_GND_CTRL = false;
      Z_ATR_CTRL = false;
      Z_VENT_CTRL = false;
      VENT_GND_CTRL = false;
      FRONTEND_CTRL = false;
      VENT_PACE_CTRL = true;
      VPW_delay = Vent_pulse_width;
    state VVIR_DischargeC21_ChargeC22
      entry:
      PACE_GND_CTRL = true;
      VENT_PACE_CTRL = false;
      Z_VENT_CTRL = false;
      Z_ATR_CTRL = false;
      ATR_PACE_CTRL = false;
      ATR_GND_CTRL = false;
      VENT_GND_CTRL = true;
      PACE_AMP = Vent_amplitude;
      PACE_CHARGE_CTRL = true;
    VVIR_DischargeC21_ChargeC22 -> VVIR.VRP [order 1] : [VENT_CMP_DETECT==true]
        | {VPW_delay = 0;}
    VVIR_PACE_VENT -> VVIR.VRP : after(Vent_pulse_width, msec)
    VVIR.VRP -> VVIR_DischargeC21_ChargeC22 : after(VRP, msec)
    VVIR_DischargeC21_ChargeC22 -> VVIR_PACE_VENT [order 2] : after(Period_R-VRP-VPW_delay, msec)
  state DOO [group]
    state DOO_DischargeC21V_ChargeC22A
      entry:
      PACE_GND_CTRL = true;
      VENT_PACE_CTRL = false;
      Z_VENT_CTRL = false;
      Z_ATR_CTRL = false;
      ATR_PACE_CTRL = false;
      ATR_GND_CTRL = false;
      VENT_GND_CTRL = true;
      PACE_AMP = Atrial_amplitude;
      PACE_CHARGE_CTRL = true;
    state DOO_PACE_ATRIUM
      entry:
      PACE_CHARGE_CTRL = false;
      PACE_GND_CTRL = true;
      VENT_PACE_CTRL = false;
      VENT_GND_CTRL = false;
      Z_VENT_CTRL = false;
      Z_ATR_CTRL = false;
      ATR_GND_CTRL = false;
      ATR_PACE_CTRL = true;
    state DOO_DischargeC21A_ChargeC22V
      entry:
      PACE_GND_CTRL = true;
      ATR_PACE_CTRL = false;
      Z_ATR_CTRL = false;
      Z_VENT_CTRL = false;
      VENT_PACE_CTRL = false;
      VENT_GND_CTRL = false;
      ATR_GND_CTRL = true;
      PACE_AMP = Vent_amplitude;
      PACE_CHARGE_CTRL = true;
    state DOO_PACE_VENT
      entry:
      PACE_CHARGE_CTRL = false;
      PACE_GND_CTRL = true;
      ATR_PACE_CTRL = false;
      ATR_GND_CTRL = false;
      Z_ATR_CTRL = false;
      Z_VENT_CTRL = false;
      VENT_GND_CTRL = false;
      VENT_PACE_CTRL = true;
    DOO_DischargeC21V_ChargeC22A -> DOO_PACE_ATRIUM [order 1] : after(Lower_period-(AV_delay+Vent_pulse_width), msec)
    DOO_PACE_ATRIUM -> DOO_DischargeC21A_ChargeC22V : after(Atrial_pulse_width, msec)
    DOO_PACE_VENT -> DOO_DischargeC21V_ChargeC22A : after(Vent_pulse_width, msec)
    DOO_DischargeC21A_ChargeC22V -> DOO_PACE_VENT : after(AV_delay - Atrial_pulse_width, msec)
  state DOOR [group]
    state DOOR_DischargeC21V_ChargeC22A
      entry:
      PACE_GND_CTRL = true;
      VENT_PACE_CTRL = false;
      Z_VENT_CTRL = false;
      Z_ATR_CTRL = false;
      ATR_PACE_CTRL = false;
      ATR_GND_CTRL = false;
      VENT_GND_CTRL = true;
      PACE_AMP = Atrial_amplitude;
      PACE_CHARGE_CTRL = true;
    state DOOR_PACE_ATRIUM
      entry:
      PACE_CHARGE_CTRL = false;
      PACE_GND_CTRL = true;
      VENT_PACE_CTRL = false;
      VENT_GND_CTRL = false;
      Z_VENT_CTRL = false;
      Z_ATR_CTRL = false;
      ATR_GND_CTRL = false;
      ATR_PACE_CTRL = true;
    state DOOR_DischargeC21A_ChargeC22V
      entry:
      PACE_GND_CTRL = true;
      ATR_PACE_CTRL = false;
      Z_ATR_CTRL = false;
      Z_VENT_CTRL = false;
      VENT_PACE_CTRL = false;
      VENT_GND_CTRL = false;
      ATR_GND_CTRL = true;
      PACE_AMP = Vent_amplitude;
      PACE_CHARGE_CTRL = true;
    state DOOR_PACE_VENT
      entry:
      PACE_CHARGE_CTRL = false;
      PACE_GND_CTRL = true;
      ATR_PACE_CTRL = false;
      ATR_GND_CTRL = false;
      Z_ATR_CTRL = false;
      Z_VENT_CTRL = false;
      VENT_GND_CTRL = false;
      VENT_PACE_CTRL = true;
    DOOR_DischargeC21V_ChargeC22A -> DOOR_PACE_ATRIUM [order 1] : after(Period_R-(AV_delay+Vent_pulse_width), msec)
    DOOR_PACE_VENT -> DOOR_DischargeC21V_ChargeC22A : after(Vent_pulse_width, msec)
    DOOR_PACE_ATRIUM -> DOOR_DischargeC21A_ChargeC22V : after(Atrial_pulse_width, msec)
    DOOR_DischargeC21A_ChargeC22V -> DOOR_PACE_VENT : after(AV_delay - Atrial_pulse_width, msec)
  AOOR_DischargeC21_ChargeC22 -> STANDBY [order 2] : [MODE~=6]
  VOOR_DischargeC21_ChargeC22 -> STANDBY [order 2] : [MODE~=7]
  VVIR_DischargeC21_ChargeC22 -> STANDBY [order 3] : [MODE~=9]
  AAIR_DischargeC21_ChargeC22 -> STANDBY [order 3] : [MODE~=8]
  STANDBY -> AAIR_DischargeC21_ChargeC22 [order 9] : [MODE==8]
      | {LED_red=false}
  STANDBY -> VVIR_DischargeC21_ChargeC22 [order 11] : [MODE==9]
      | {LED_red=false}
  STANDBY -> DOOR_DischargeC21V_ChargeC22A [order 10] : [MODE==10]
      | {LED_red=false}
  STANDBY -> AOOR_DischargeC21_ChargeC22 [order 7] : [MODE==6]
      | {LED_red=false}
  STANDBY -> VOOR_DischargeC21_ChargeC22 [order 8] : [MODE==7]
      | {LED_red=false}
  VVI_DischargeC21_ChargeC22 -> STANDBY [order 3] : [MODE~=4]
  VOO_DischargeC21_ChargeC22 -> STANDBY [order 2] : [MODE~=2]
  STANDBY -> DOO_DischargeC21V_ChargeC22A [order 6] : [MODE==5]
      | {LED_red=false}
  DOOR_DischargeC21V_ChargeC22A -> STANDBY [order 2] : [MODE~=10]
  AOO_DischargeC21_ChargeC22 -> STANDBY [order 2] : [MODE~=1]
  AAI_DischargeC21_ChargeC22 -> STANDBY [order 3] : [MODE~=3]
  DOO_DischargeC21V_ChargeC22A -> STANDBY [order 2] : [MODE~=5]
  STANDBY -> AAI_DischargeC21_ChargeC22 [order 3] : [MODE==3]
      | {LED_red=false}
  STANDBY -> VVI_DischargeC21_ChargeC22 [order 5] : [MODE==4]
      | {LED_red=false}
  STANDBY -> VOO_DischargeC21_ChargeC22 [order 4] : [MODE==2]
      | {LED_red=false}
  STANDBY -> AOO_DischargeC21_ChargeC22 [order 2] : [MODE==1]
      | {LED_red=false}
  (default) -> STANDBY
  STANDBY -> STANDBY [order 1] : [MODE==0 || Lower_rate_limit>Upper_rate_limit]
  data: PACE_AMP output double; MODE input uint8; Atrial_amplitude input double; Vent_amplitude input double; Lower_period input uint16; Lower_rate_limit input uint16; Upper_rate_limit input uint16; Atrial_pulse_width input uint16; PACE_CHARGE_CTRL output boolean; ATR_PACE_CTRL output boolean; ATR_GND_CTRL output boolean; Z_ATR_CTRL output boolean; VENT_PACE_CTRL output boolean; VENT_GND_CTRL output boolean; Z_VENT_CTRL output boolean; PACE_GND_CTRL output boolean; FRONTEND_CTRL output boolean; LED_red output boolean; LED_green output boolean; LED_blue output boolean; Vent_pulse_width input uint16; ARP input uint16; VRP input uint16; AV_delay input uint16; ATR_CMP_DETECT input boolean; VENT_CMP_DETECT input boolean; APW_delay local uint16; VPW_delay local uint16; Period_R input uint16

== matlab function Pacemaker_model_assgn2_2019a/RATE_ADAPTIVE/get_Steps/MATLAB Function ==
  data: LRL input; dY output; MSR input; RF input; dT input; time input
function dY = getStep(LRL, MSR, RF, dT, time)
dY = ((RF/8)*(MSR-LRL)/(time*1000))*dT;

== matlab function Pacemaker_model_assgn2_2019a/RATE_ADAPTIVE/get_Thresh_Vals/MATLAB Function ==
  data: level input; vals output; max_accel input
function vals = getActThresh(level, max_accel)
if level==1
    AT = 0.4;
elseif level==3
    AT = 0.8;
elseif level==4
    AT = 1.0;
else
    AT = 0.6;
end
    AT1 = (max_accel - AT)*(1/3) + AT;
    AT2 = (max_accel - AT)*(2/3) + AT;
vals = [AT AT1 AT2];
